simulink model "spring_mass_dumper"  (R2019b)
settings: Solver=VariableStepAuto  StartTime=0.0  StopTime=100  RelTol=1e-13
settings Model: Creator=adity  LastModifiedBy=adity

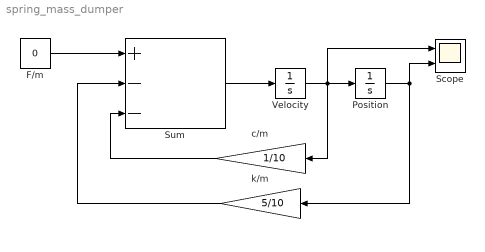
== system spring_mass_dumper ==
  "F/m " : Constant  Value=0
  Position : Integrator
  Scope : Scope  NumInputPorts=2
  Sum : Sum  Inputs=+--
  Velocity : Integrator  InitialCondition=8
  c/m : Gain  Gain=1/10
  k/m : Gain  Gain=5/10
  wires:
  Velocity/1 -> Scope/1, c/m/1, Position/1
  Sum/1 -> Velocity/1
  Position/1 -> k/m/1, Scope/2
  k/m/1 -> Sum/2
  c/m/1 -> Sum/3
  "F/m "/1 -> Sum/1
